simulink model "rtlab_simple_io"  (Simulink 7.8)
settings: Solver=ode3  StartTime=0.0  StopTime=Inf  FixedStep=1e-5  RelTol=1e-3
libraries: rtlab x2, opal_lib x1
Description:
  | Model of a simple control system for use iin training.
settings Model: Creator=Paul Baracos  LastModifiedBy=sfrank1  BufferReuse=off
settings DataIOCC: SaveOutput=off  SaveTime=off  SignalLoggingName=sigsOut
settings OptimizationCC: BlockReduction=off  BooleanDataType=off  InlineInvariantSignals=on  OptimizeBlockIOStorage=off  BufferReuse=off  ExpressionFolding=off  LocalBlockOutputs=off  InitFltsAndDblsToZero=on
settings DebuggingCC: SaveWithParameterizedLinksMsg=none  SignalResolutionControl=TryResolveAllWithWarning  SolverPrmCheckMsg=none  MultiTaskDSMMsg=warning  MultiTaskCondExecSysMsg=none  FcnCallInpInsideContextMsg=Use local settings  StrictBusMsg=None
settings HardwareCC: TargetUnknown=on
settings RTWCC: IncludeERTFirstTime=on
settings GRTTargetCC: TargetFcnLib=ansi_tfl_tmw.mat

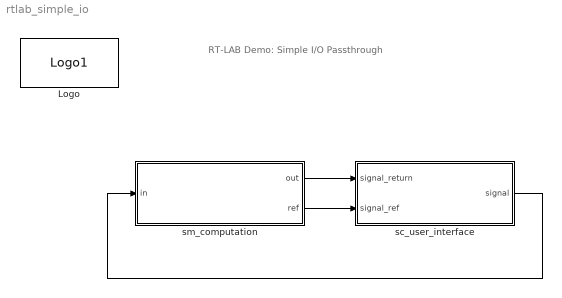
== system rtlab_simple_io ==
  note: RT-LAB Demo: Simple I/O Passthrough
  Logo : opal_lib/Logo1  vide=[]
  sc_user_interface : Subsystem
  sm_computation : Subsystem
  wires:
  sc_user_interface/1(signal) -> sm_computation/1(in)
  sm_computation/1(out) -> sc_user_interface/1(signal_return)
  sm_computation/2(ref) -> sc_user_interface/2(signal_ref)

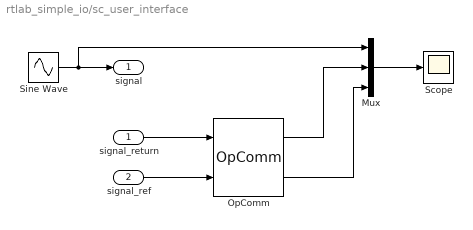
== system rtlab_simple_io/sc_user_interface ==
  signal_return : Inport
  signal_ref : Inport  Port=2
  Mux : Mux  Inputs=3
  OpComm : rtlab/OpComm  nbport=2  groupe_acq=1  subsys_rate=0  st=0  Synchronization=on  Interpolation=on  Threshold=1.0  Missed_Data=off  Sim_Time=off  Samples=off  dynSigOut=off  from_console=0  warning_done=off  writeOpCommFile=off  Offset=off
  Scope : Scope
      settings: YMin=-1  YMax=1
  Sine Wave : Sin  SampleTime=0
  signal : Outport
  wires:
  Sine Wave/1 -> signal/1, Mux/1
  Mux/1 -> Scope/1
  signal_return/1 -> OpComm/1
  OpComm/1 -> Mux/2
  signal_ref/1 -> OpComm/2
  OpComm/2 -> Mux/3

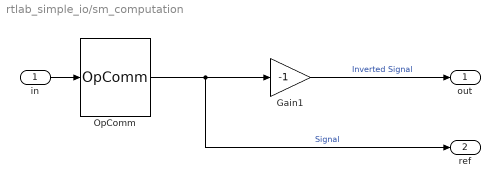
== system rtlab_simple_io/sm_computation ==
  in : Inport
  Gain1 : Gain  Gain=-1  SaturateOnIntegerOverflow=on  OutDataTypeStr=Inherit: Same as input  ParamDataTypeStr=Inherit: Same as input
  OpComm : rtlab/OpComm  nbport=1  groupe_acq=1  subsys_rate=0  st=0  Synchronization=on  Interpolation=on  Threshold=1.0  Missed_Data=off  Sim_Time=off  Samples=off  dynSigOut=off  from_console=1  warning_done=off  writeOpCommFile=off  Offset=off
  out : Outport
  ref : Outport  Port=2
  wires:
  in/1 -> OpComm/1
  OpComm/1 -> Gain1/1, ref/1  "Signal"
  Gain1/1 -> out/1  "Inverted Signal"
